simulink model "fip"  (R2019a)
settings: Solver=VariableStepAuto  StartTime=0.0  StopTime=T  RelTol=1e-3
values from neighbouring files (symbols this model uses):
  g = 9.81    [fip.m]    (also in fip_init.m)
  h = 0.01    [fip_init.m]    (also in rk4.m = (b - a) / n)
  L = 1    [fip.m]    (also in fip_init.m)
  x0 = [0.1; -0.2; 0.5]    [fip_init.m]
  xd0 = [0; 0; 0]    [fip_init.m]
undefined symbols (not defined in the file or in its folder): K_x, K_y, K_z
settings Model: Creator=martinbrandt  LastModifiedBy=martinbrandt

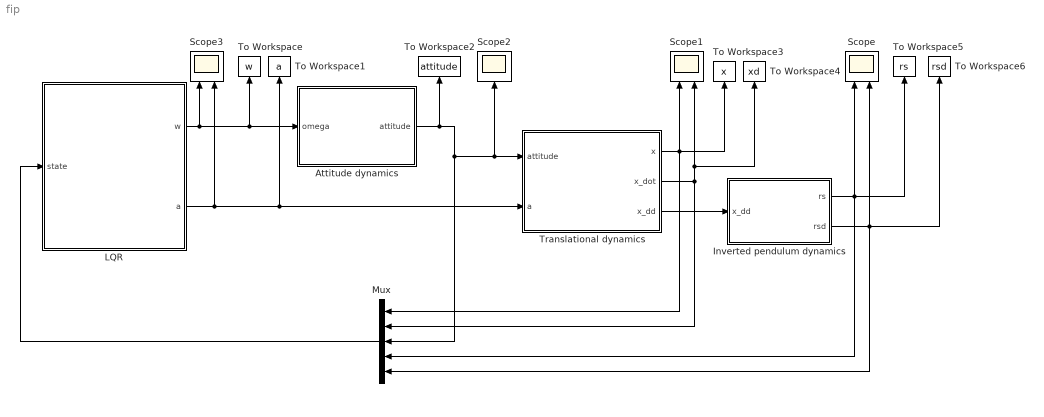
== system fip ==
  Attitude dynamics : Subsystem
  "Inverted pendulum dynamics " : Subsystem
  LQR : Subsystem
  Mux : Mux  Inputs=5
  Scope : Scope  NumInputPorts=2
  Scope1 : Scope  NumInputPorts=2
  Scope2 : Scope
  Scope3 : Scope  NumInputPorts=2
  To Workspace : ToWorkspace  VariableName=w  SaveFormat=Timeseries  SampleTime=h
  To Workspace1 : ToWorkspace  VariableName=a  SaveFormat=Timeseries  SampleTime=h
  To Workspace2 : ToWorkspace  VariableName=attitude  SaveFormat=Timeseries  SampleTime=h
  To Workspace3 : ToWorkspace  VariableName=x  SaveFormat=Timeseries  SampleTime=h
  To Workspace4 : ToWorkspace  VariableName=xd  SaveFormat=Timeseries  SampleTime=h
  To Workspace5 : ToWorkspace  VariableName=rs  SaveFormat=Timeseries  SampleTime=h
  To Workspace6 : ToWorkspace  VariableName=rsd  SaveFormat=Timeseries  SampleTime=h
  Translational dynamics : Subsystem
  wires:
  Translational dynamics/3(x_dd) -> "Inverted pendulum dynamics "/1(x_dd)
  Translational dynamics/1(x) -> To Workspace3/1, Mux/1, Scope1/1
  Translational dynamics/2(x_dot) -> To Workspace4/1, Scope1/2, Mux/2
  LQR/2(a) -> Translational dynamics/2(a), To Workspace1/1, Scope3/2
  LQR/1(w) -> Attitude dynamics/1(omega), To Workspace/1, Scope3/1
  Attitude dynamics/1(attitude) -> To Workspace2/1, Mux/3, Scope2/1, Translational dynamics/1(attitude)
  "Inverted pendulum dynamics "/2("rsd ") -> To Workspace6/1, Scope/2, Mux/5
  "Inverted pendulum dynamics "/1(rs) -> To Workspace5/1, Scope/1, Mux/4
  Mux/1 -> LQR/1(state)

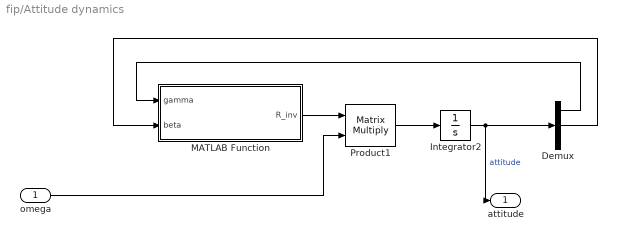
== system fip/Attitude dynamics ==
  omega : Inport
  Demux : Demux  Outputs=3
  Integrator2 : Integrator
  MATLAB Function : MATLAB Function  TreatAsAtomicUnit=on
  Product1 : Product  Multiplication=Matrix(*)
  attitude : Outport
  wires:
  MATLAB Function/1(R_inv) -> Product1/1
  omega/1 -> Product1/2
  Integrator2/1 -> attitude/1, Demux/1  "attitude"
  Demux/2 -> MATLAB Function/2(beta)
  Product1/1 -> Integrator2/1
  Demux/1 -> MATLAB Function/1(gamma)

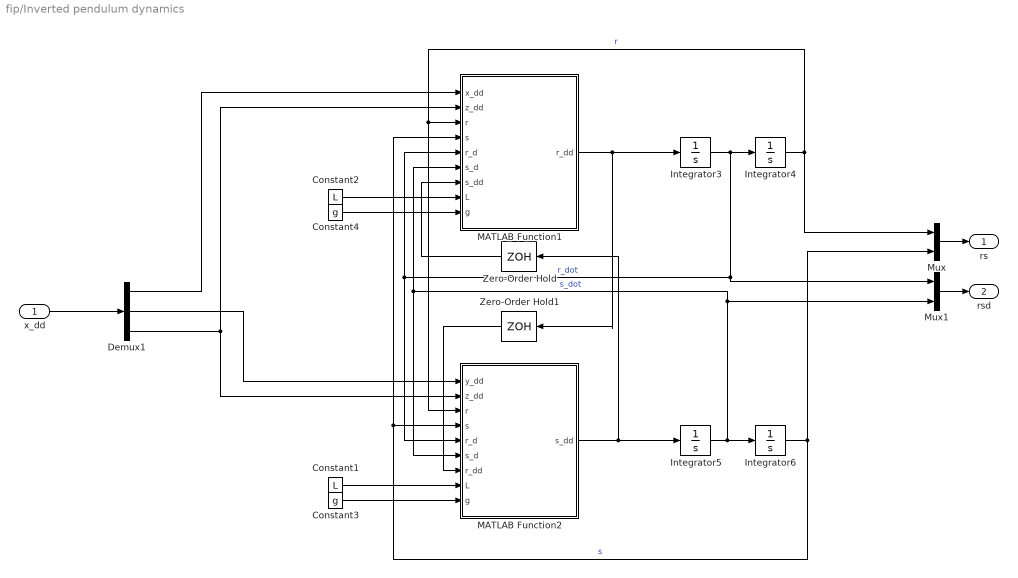
== system fip/Inverted pendulum dynamics  ==
  x_dd : Inport
  Constant1 : Constant  Value=L
  Constant2 : Constant  Value=L
  Constant3 : Constant  Value=g
  Constant4 : Constant  Value=g
  Demux1 : Demux  Outputs=3
  Integrator{3..6} (4 alike) : Integrator
  MATLAB Function1 : MATLAB Function  TreatAsAtomicUnit=on
  MATLAB Function2 : MATLAB Function  TreatAsAtomicUnit=on
  Mux : Mux  Inputs=2
  Mux1 : Mux  Inputs=2
  Zero-Order Hold : ZeroOrderHold  SampleTime=0.0001
  Zero-Order Hold1 : ZeroOrderHold  SampleTime=0.0001
  rs : Outport
  "rsd " : Outport  Port=2
  wires:
  MATLAB Function2/1(s_dd) -> Zero-Order Hold/1, Integrator5/1
  x_dd/1 -> Demux1/1
  Demux1/2 -> MATLAB Function2/1(y_dd)
  Demux1/3 -> MATLAB Function2/2(z_dd), MATLAB Function1/2(z_dd)
  Demux1/1 -> MATLAB Function1/1(x_dd)
  MATLAB Function1/1(r_dd) -> Zero-Order Hold1/1, Integrator3/1
  Integrator6/1 -> Mux/2, MATLAB Function1/4(s), MATLAB Function2/4(s)  "s"
  Integrator3/1 -> Mux1/1, MATLAB Function1/5(r_d), MATLAB Function2/5(r_d), Integrator4/1  "r_dot"
  Integrator5/1 -> Mux1/2, MATLAB Function2/6(s_d), MATLAB Function1/6(s_d), Integrator6/1  "s_dot"
  Integrator4/1 -> Mux/1, MATLAB Function2/3(r), MATLAB Function1/3(r)  "r"
  Constant1/1 -> MATLAB Function2/8(L)
  Constant3/1 -> MATLAB Function2/9(g)
  Constant2/1 -> MATLAB Function1/8(L)
  Constant4/1 -> MATLAB Function1/9(g)
  Zero-Order Hold/1 -> MATLAB Function1/7(s_dd)
  Zero-Order Hold1/1 -> MATLAB Function2/7(r_dd)
  Mux/1 -> rs/1
  Mux1/1 -> "rsd "/1

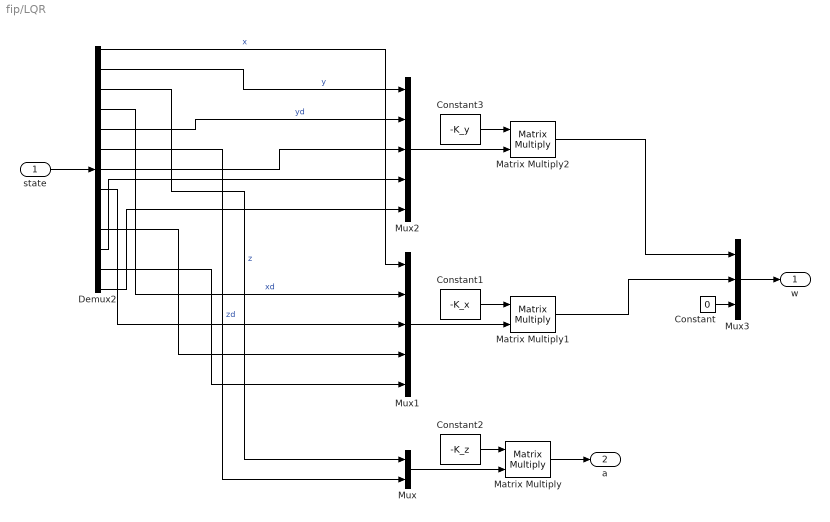
== system fip/LQR ==
  state : Inport
  Constant : Constant  Value=0
  Constant1 : Constant  Value=-K_x  VectorParams1D=off
  Constant2 : Constant  Value=-K_z  VectorParams1D=off
  Constant3 : Constant  Value=-K_y  VectorParams1D=off
  Demux2 : Demux  Outputs=13
  Matrix Multiply : Product  Multiplication=Matrix(*)
  Matrix Multiply1 : Product  Multiplication=Matrix(*)
  Matrix Multiply2 : Product  Multiplication=Matrix(*)
  Mux : Mux  Inputs=2
  Mux1 : Mux  Inputs=5
  Mux2 : Mux  Inputs=5
  Mux3 : Mux  Inputs=3
  w : Outport
  a : Outport  Port=2
  wires:
  Matrix Multiply/1 -> a/1
  Demux2/8 -> Mux1/3
  Mux1/1 -> Matrix Multiply1/2
  Demux2/3 -> Mux/1  "z"
  Demux2/5 -> Mux2/2  "yd"
  Demux2/2 -> Mux2/1  "y"
  Demux2/6 -> Mux/2  "zd"
  Demux2/1 -> Mux1/1  "x"
  Demux2/4 -> Mux1/2  "xd"
  Constant2/1 -> Matrix Multiply/1
  Mux/1 -> Matrix Multiply/2
  Constant1/1 -> Matrix Multiply1/1
  Constant3/1 -> Matrix Multiply2/1
  Mux2/1 -> Matrix Multiply2/2
  Demux2/7 -> Mux2/3
  Demux2/10 -> Mux1/4
  Demux2/11 -> Mux2/4
  Demux2/12 -> Mux1/5
  Demux2/13 -> Mux2/5
  Constant/1 -> Mux3/3
  Matrix Multiply1/1 -> Mux3/2
  Matrix Multiply2/1 -> Mux3/1
  Mux3/1 -> w/1
  state/1 -> Demux2/1

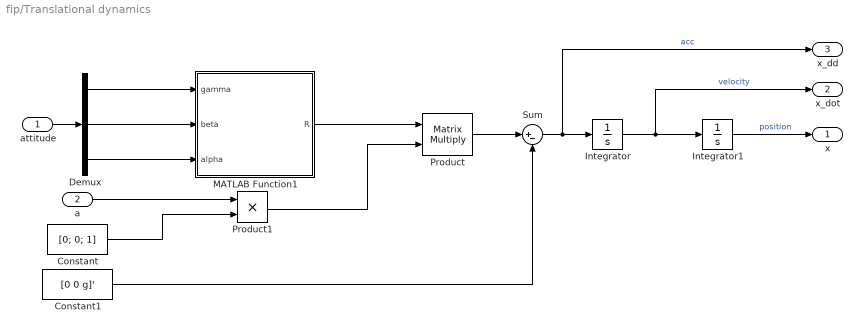
== system fip/Translational dynamics ==
  attitude : Inport
  a : Inport  Port=2
  Constant : Constant  Value=[0; 0; 1]  VectorParams1D=off
  Constant1 : Constant  Value=[0 0 g]'  VectorParams1D=off
  Demux : Demux  Outputs=3
  Integrator : Integrator  InitialCondition=xd0
  Integrator1 : Integrator  InitialCondition=x0
  MATLAB Function1 : MATLAB Function  TreatAsAtomicUnit=on
  Product : Product  Multiplication=Matrix(*)
  Product1 : Product
  Sum : Sum  Inputs=|+-
  x : Outport
  x_dot : Outport  Port=2
  x_dd : Outport  Port=3
  wires:
  Demux/1 -> MATLAB Function1/1(gamma)
  MATLAB Function1/1(R) -> Product/1
  Demux/2 -> MATLAB Function1/2(beta)
  Integrator1/1 -> x/1  "position"
  Constant1/1 -> Sum/2
  Integrator/1 -> x_dot/1, Integrator1/1  "velocity"
  a/1 -> Product1/1
  Demux/3 -> MATLAB Function1/3(alpha)
  Sum/1 -> x_dd/1, Integrator/1  "acc"
  Product/1 -> Sum/1
  Constant/1 -> Product1/2
  Product1/1 -> Product/2
  attitude/1 -> Demux/1

== matlab function fip/Translational dynamics/MATLAB Function1 ==
  data: gamma input; R output; beta input; alpha input
function R = R_vo(gamma, beta, alpha)
R_z = [cos(alpha) -sin(alpha) 0; sin(alpha) cos(alpha) 0; 0 0 1];
R_y = [cos(beta) 0 sin(beta); 0 1 0; -sin(beta) 0 cos(beta)];
R_x = [1 0 0; 0 cos(gamma) -sin(gamma); 0 sin(gamma) cos(gamma)];
R = R_z * R_y * R_x;

== matlab function fip/Attitude dynamics/MATLAB Function ==
  data: gamma input; R_inv output; beta input
function R_inv = R_euler_rates(gamma, beta)
R_inv = inv([cos(beta) * cos(gamma) -sin(gamma) 0; cos(beta) * sin(gamma) cos(gamma) 0; -sin(beta) 0 1]);

== matlab function fip/Inverted pendulum dynamics /MATLAB Function2 ==
  data: y_dd input; s_dd output; z_dd input; r input; s input; r_d input; s_d input; r_dd input; L input; g input
function s_dd = f_s_dd(y_dd, z_dd, r, s, r_d, s_d, r_dd, L, g)
    zeta = sqrt(L^2 - r^2 - s^2);
    s_dd = (-s^4 * y_dd - (L^2 - r^2)^2 * y_dd - 2 * s^2 * (r * r_d * s_d + (-L^2 + r^2) * y_dd) ...
    + s^3 * (r_d^2 + r * r_dd^2 - zeta * (g + z_dd)) ...
    + s * (-L^2 * r * r_dd + r^3 * r_dd + r^2 * (s_d^2 - zeta * (g + z_dd)) ...
    + L^2 * (-r_d^2 - s_d^2 + zeta * (g + z_dd)))) / ((L^2 - r^2) * zeta^2);
end

== matlab function fip/Inverted pendulum dynamics /MATLAB Function1 ==
  data: x_dd input; r_dd output; z_dd input; r input; s input; r_d input; s_d input; s_dd input; L input; g input
function r_dd = f_r_dd(x_dd, z_dd, r, s, r_d, s_d, s_dd, L, g)
    zeta = sqrt(L^2 - r^2 - s^2);
    r_dd = (-r^4 * x_dd - (L^2 - s^2)^2 * x_dd - 2 * r^2 * (s * r_d * s_d + (-L^2 + s^2) * x_dd) ...
    + r^3 * (s_d^2 + s * s_dd^2 - zeta * (g + z_dd)) ...
    + r * (-L^2 * s * s_dd + s^3 * s_dd + s^2 * (r_d^2 - zeta * (g + z_dd)) ...
    + L^2 * (-r_d^2 - s_d^2 + zeta * (g + z_dd)))) / ((L^2 - s^2) * zeta^2);
end
